simulink model "sat_orbit_orientation_prop_only_SIM"  (R2019b)
settings: Solver=VariableStepAuto  StartTime=0.0  StopTime=15000.0  MaxStep=0.05  RelTol=1e-8
libraries: simulink x1
settings Model: Creator=Hector  LastModifiedBy=Hector
settings SolverCC: AlgebraicLoopSolver=LineSearch
settings DebuggingCC: AlgebraicLoopMsg=none

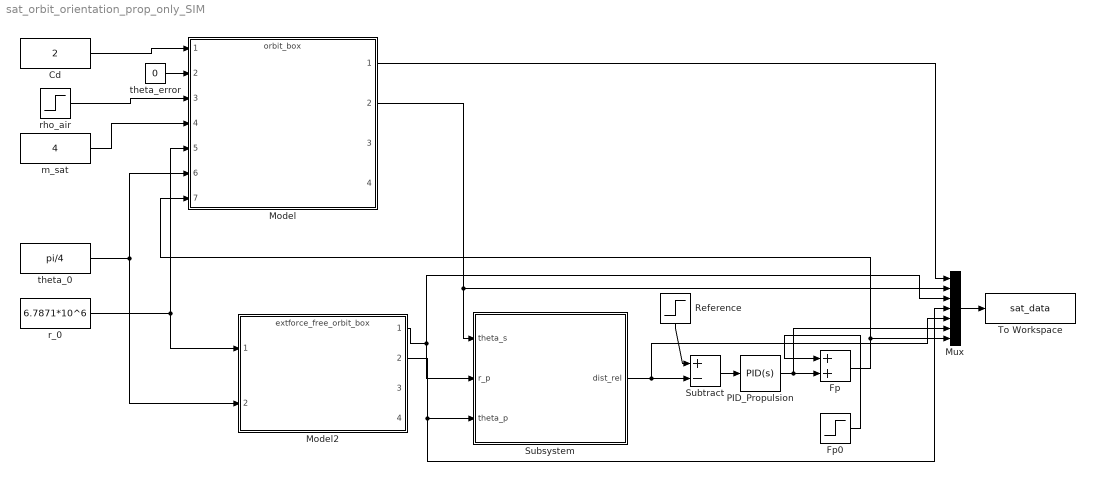
== system sat_orbit_orientation_prop_only_SIM ==
  Cd : Constant  Value=2
  Fp : Sum
  Fp0 : Step  Time=0  Before=1.2861*10^(-6)  After=1.2861*10^(-6)  SampleTime=1
  Model : ModelReference  ModelNameDialog=orbit_box.slx  SimulationMode=Normal  ModelReferenceVersion=1.37
  Model2 : ModelReference  ModelNameDialog=extforce_free_orbit_box.slx  SimulationMode=Normal  ModelReferenceVersion=1.35
  Mux : Mux  Inputs=7
  PID_Propulsion : simulink/Continuous/PID Controller  Controller=PID  Form=Parallel  TimeDomain=Continuous-time  SampleTime=-1  IntegratorMethod=Forward Euler  FilterMethod=Forward Euler  ControllerParametersSource=internal  P=2.11519715784155e-06  I=1.28628982869464e-10  D=0.00754921104528398  UseFilter=on  N=0.228565595208321  TunerSelectOption=Transfer Function Based (PID Tuner App)  InitialConditionSource=internal  InitialConditionForIntegrator=0  InitialConditionForFilter=0  DifferentiatorICPrevScaledInput=0  ExternalReset=none  TrackingMode=off  Kt=1  LimitOutput=off  UpperSaturationLimit=.05e-03  LowerSaturationLimit=0  LinearizeAsGain=off  AntiWindupMode=none  Kb=1  POutMin=[]  POutMax=[]  IOutMin=[]  IOutMax=[]  DOutMin=[]  DOutMax=[]  NOutMin=[]  NOutMax=[]  SumOutMin=[]  SumOutMax=[]  SaturationOutMin=[]  SaturationOutMax=[]  PParamMin=[]  PParamMax=[]  IParamMin=[]  IParamMax=[]  DParamMin=[]  DParamMax=[]  NParamMin=[]  NParamMax=[]  KbParamMin=[]  KbParamMax=[]  KtParamMin=[]  KtParamMax=[]  KbOutMin=[]  KbOutMax=[]  KtOutMin=[]  KtOutMax=[]  IntegratorOutMin=[]  IntegratorOutMax=[]  FilterOutMin=[]  FilterOutMax=[]  SumI1OutMin=[]  SumI1OutMax=[]  SumI2OutMin=[]  SumI2OutMax=[]  SumI3OutMin=[]  SumI3OutMax=[]  SumI4OutMin=[]  SumI4OutMax=[]  SumDOutMin=[]  SumDOutMax=[]  DifferentiatorOutMin=[]  DifferentiatorOutMax=[]  FilterDiffOutCoefMin=[]  FilterDiffOutCoefMax=[]  ReciprocalOutMin=[]  ReciprocalOutMax=[]  SumDenOutMin=[]  SumDenOutMax=[]  SumNumOutMin=[]  SumNumOutMax=[]  DivideOutMin=[]  DivideOutMax=[]  IntegratorContinuousStateAttributes=''  IntegratorStateMustResolveToSignalObject=off  IntegratorRTWStateStorageClass=Auto  FilterContinuousStateAttributes=''  FilterStateMustResolveToSignalObject=off  FilterRTWStateStorageClass=Auto  ParallelPVariant=InternalParameters  IdealPVariant=Disabled  IVariant=InternalParameters  DVariant=InternalParameters  IntegratorVariant=Continuous  SatVariant=Disabled  AWVariant=Passthrough  PCopyVariant=Disabled  TRVariant=Disabled  FdbkBlocksVariant=Forward  IdealPFdbkVariant=Disabled  SatFdbkVariant=Disabled  DerivativeFilterVariant=ContFilter  NVariant=InternalParameters  NCopyVariant=Disabled  FilterICVariant=InternalICsFilter  IntegratorICVariant=InternalICs  ExternalResetVariant=Disabled  TRSumVariant=Passthrough  SumFdbkVariant=Disabled  SumVariant=Sum_PID
  "Reference " : Step  Time=0  Before=0.02  After=0.02  SampleTime=1
  Subsystem : Subsystem
  Subtract : Sum  Inputs=+-
  To Workspace : ToWorkspace  VariableName=sat_data  SampleTime=-1
  m_sat : Constant  Value=4
  r_0 : Constant  Value=6.7871*10^6
  rho_air : Step  Time=0  Before=0.219*10^(-11)  After=0.219*10^(-11)  SampleTime=0
  theta_0 : Constant  Value=pi/4
  theta_error : Constant  Value=0
  wires:
  Cd/1 -> Model/1
  rho_air/1 -> Model/3
  m_sat/1 -> Model/4
  r_0/1 -> Model/5, Model2/1
  theta_0/1 -> Model/6, Model2/2
  Model/2 -> Mux/2, Subsystem/1(theta_s)
  Model/1 -> Mux/1
  Mux/1 -> To Workspace/1
  Model2/1 -> Mux/3, Subsystem/2(r_p)
  Model2/2 -> Mux/4, Subsystem/3(theta_p)
  Fp0/1 -> Fp/1
  PID_Propulsion/1 -> Mux/6, Fp/2
  Fp/1 -> Model/7, Mux/7
  theta_error/1 -> Model/2
  Subsystem/1(dist_rel) -> Mux/5, Subtract/2
  Subtract/1 -> PID_Propulsion/1
  "Reference "/1 -> Subtract/1

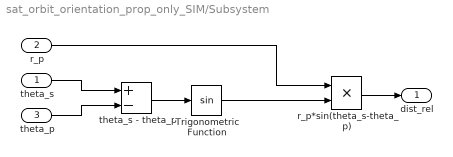
== system sat_orbit_orientation_prop_only_SIM/Subsystem ==
  theta_s : Inport
  r_p : Inport  Port=2
  theta_p : Inport  Port=3
  Trigonometric Function : Trigonometry
  r_p*sin(theta_s-theta_p) : Product
  theta_s - theta_p : Sum  Inputs=+-
  dist_rel : Outport
  wires:
  r_p/1 -> r_p*sin(theta_s-theta_p)/1
  theta_s/1 -> theta_s - theta_p/1
  theta_p/1 -> theta_s - theta_p/2
  theta_s - theta_p/1 -> Trigonometric Function/1
  r_p*sin(theta_s-theta_p)/1 -> dist_rel/1
  Trigonometric Function/1 -> r_p*sin(theta_s-theta_p)/2
